simulink model "ODEPendulo"  (R2021b)
settings: Solver=VariableStepAuto  StartTime=0.0  StopTime=1.5  RelTol=1e-3
values from neighbouring files (symbols this model uses):
  g = 9.8    [regresionpendulo_1_gr.m]    (also in regresionpendulo_1_pq.m)
  l = 0.3    [regresionpendulo_1_gr.m]    (also in regresionpendulo_1_pq.m)
  phi = 1.57    [regresionpendulo_1_gr.m]    (also in regresionpendulo_1_pq.m)
  theta_m = (max(y_theta)-min(y_theta))/2    [regresionpendulo_1_gr.m]    (also in regresionpendulo_1_pq.m)
  Wn = sqrt(g/l)    [regresionpendulo_1_gr.m]    (also in regresionpendulo_1_pq.m)
settings Model: Creator=Federico  LastModifiedBy=Federico

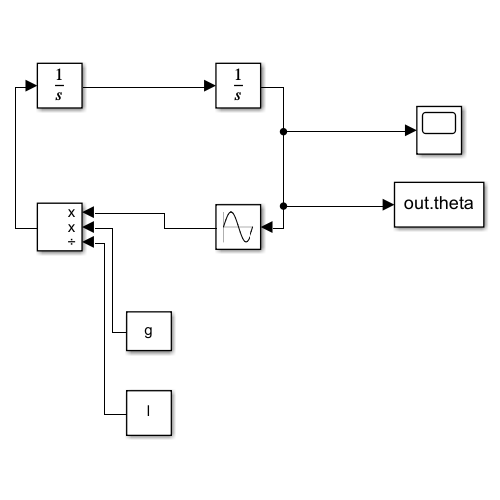
[thumbnail: Simulink's stored preview of the top-level diagram]
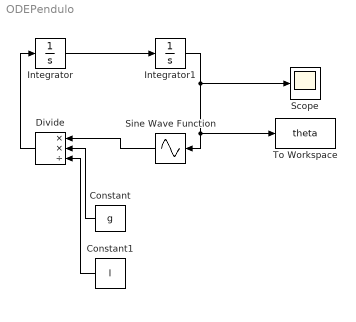
== system ODEPendulo ==
  Constant : Constant  Value=g
  Constant1 : Constant  Value=l
  Divide : Product  Inputs=**/
  Integrator : Integrator
  Integrator1 : Integrator
  Scope : Scope
  Sine Wave Function : Sin  TimeSource=Use external signal  Amplitude=theta_m  Frequency=-Wn  Phase=phi  SampleTime=0
  To Workspace : ToWorkspace  VariableName=theta  SampleTime=-1
      settings: Save2DSignal=2-D array (concatenate along first dimension)
  wires:
  Constant/1 -> Divide/2
  Constant1/1 -> Divide/3
  Sine Wave Function/1 -> Divide/1
  Divide/1 -> Integrator/1
  Integrator/1 -> Integrator1/1
  Integrator1/1 -> Scope/1, To Workspace/1, Sine Wave Function/1
